simulink model "diagram_pendulum"  (R2024a)
settings: Solver=ode45  StartTime=0.0  StopTime=10.0  RelTol=1e-3
values from neighbouring files (symbols this model uses):
  g = 9.81    [pendulum.m]
  L = 1    [pendulum.m]
  theta_0 = 179.9/180*pi    (= 3.13984732434)    [pendulum.m]
settings Model: Creator=a.brugnoli  LastModifiedBy=a.brugnoli

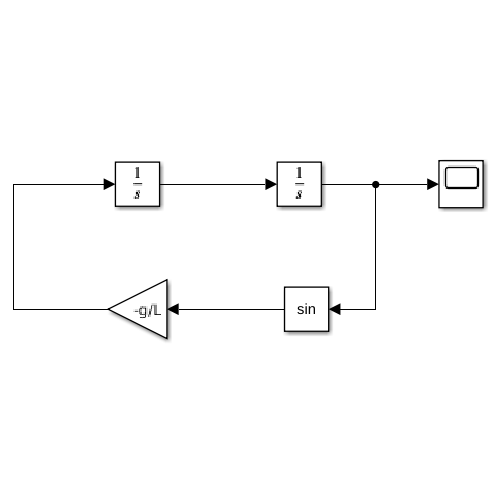
[thumbnail: Simulink's stored preview of the top-level diagram]
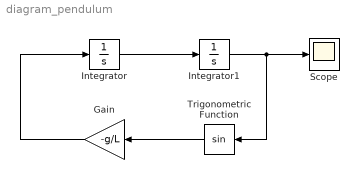
== system diagram_pendulum ==
  Gain : Gain  Gain=-g/L
  Integrator : Integrator
  Integrator1 : Integrator  InitialCondition=theta_0
  Scope : Scope
  Trigonometric Function : Trigonometry
  wires:
  Gain/1 -> Integrator/1
  Integrator/1 -> Integrator1/1
  Trigonometric Function/1 -> Gain/1
  Integrator1/1 -> Trigonometric Function/1, Scope/1
